simulink model "NoLineal_Linealizado"  (R2019a)
settings: Solver=ode4  StartTime=0.0  StopTime=0.6  FixedStep=0.001  RelTol=1e-3  EnableMultiTasking=on
settings Model: Creator=Ezequiel  LastModifiedBy=ARLUBER1
settings DataIOCC: LimitDataPoints=on  SaveFormat=Array  ReturnWorkspaceOutputs=off
settings OptimizationCC: LifeSpan=inf
settings DebuggingCC: PregeneratedLibrarySubsystemCodeDiagnostic=none  SFUnexpectedBacktrackingDiag=warning  SFNoUnconditionalDefaultTransitionDiag=warning  SFExecutionAtInitializationDiag=none  ArithmeticOperatorsInVariantConditions=warning
settings HardwareCC: ProdBitPerPointer=32  ProdBitPerSizeT=32  ProdBitPerPtrDiffT=32  ProdLargestAtomicFloat=None  ProdIntDivRoundTo=Undefined  ProdEndianess=Unspecified  ProdWordSize=32  ProdHWDeviceType=32-bit Generic
settings ModelReferenceCC: PropagateSignalLabelsOutOfModel=off
settings SFSimCC: SimUseLocalCustomCode=off
settings RTWCC: RTWUseLocalCustomCode=off
settings CodeAppCC: StateflowObjectComments=on
settings GRTTargetCC: TargetLangStandard=C89/C90 (ANSI)  GeneratePreprocessorConditionals=Disable all
settings ConfigComp: CovMetricSettings=dw  CovHtmlReporting=on  CovSaveCumulativeToWorkspaceVar=on  CovSaveSingleToWorkspaceVar=on  CovExternalEMLEnable=off

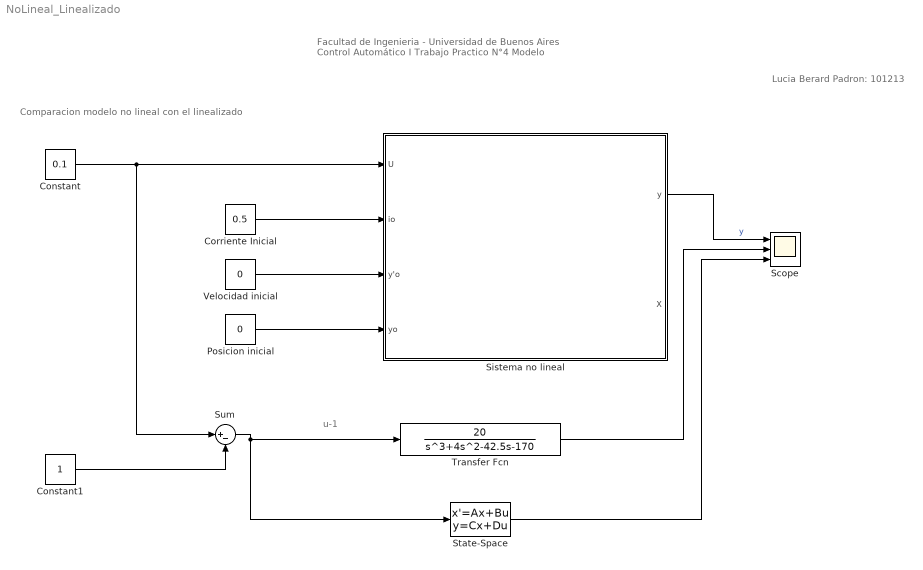
== system NoLineal_Linealizado ==
  note: Facultad de Ingenieria - Universidad de Buenos Aires
      | Control Automático I
      | Trabajo Practico N°4
      | Modelo
  note: Lucia Berard
      | Padron: 101213
  note: Comparacion modelo no lineal con el linealizado
  note: u-1
  Constant : Constant  Value=0.1
  Constant1 : Constant
  Corriente Inicial : Constant  Value=0.5
  Posicion inicial : Constant  Value=0
  Scope : Scope  NumInputPorts=3
  Sistema no lineal : Subsystem
  "State-Space " : StateSpace  A=[0 1 0;42.5 0 20;0 0 -4]  B=[0 0 1]'  C=[1 0 0]  D=0  InitialCondition=0
  Sum : Sum  Inputs=|+-
  Transfer Fcn : TransferFcn  Numerator=[20]  Denominator=[1 4 -42.5 -170]
  Velocidad inicial : Constant  Value=0
  wires:
  Corriente Inicial/1 -> Sistema no lineal/2(io)
  Velocidad inicial/1 -> Sistema no lineal/3(y'o)
  Posicion inicial/1 -> Sistema no lineal/4(yo)
  Constant/1 -> Sum/1, Sistema no lineal/1(U)
  Constant1/1 -> Sum/2
  Sum/1 -> "State-Space "/1, Transfer Fcn/1
  "State-Space "/1 -> Scope/3
  Sistema no lineal/1("y ") -> Scope/1  "y"
  Transfer Fcn/1 -> Scope/2

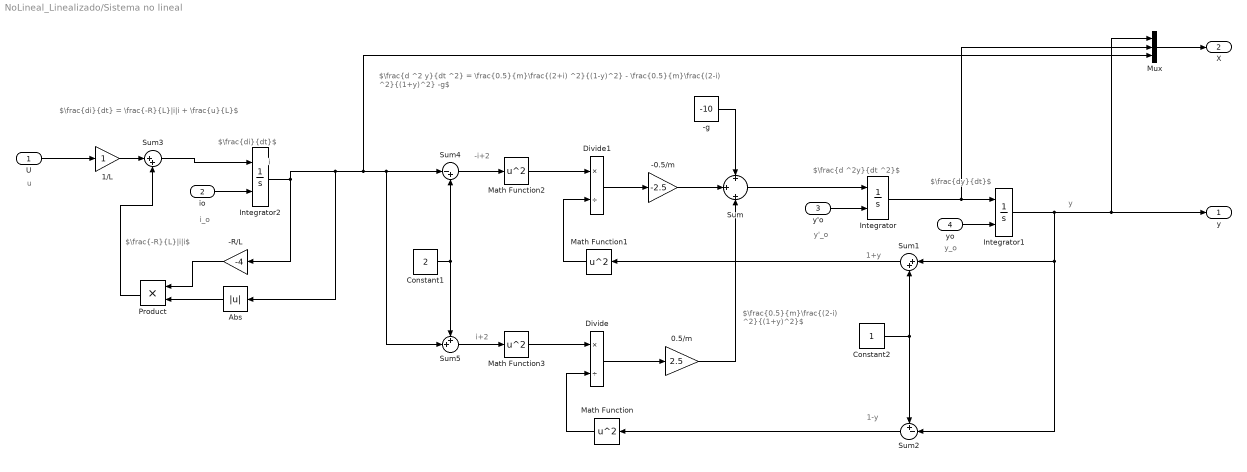
== system NoLineal_Linealizado/Sistema no lineal ==
  note: y_o
  note: y'_o
  note: i_o
  note: u
  note: i+2
  note: 1+y
  note: -i+2
  note: i
  note: y
  note: 1-y
  note: $\frac{di}{dt} = \frac{-R}{L}|i|i + \frac{u}{L}$
  note: $\frac{d ^2 y}{dt ^2} = \frac{0.5}{m}\frac{(2+i) ^2}{(1-y)^2} - \frac{0.5}{m}\frac{(2-i) ^2}{(1+y)^2} -g$
  note: $\frac{dy}{dt}$
  note: $\frac{d ^2y}{dt ^2}$
  note: $\frac{di}{dt}$
  note: $\frac{-R}{L}|i|i$
  note: $\frac{0.5}{m}\frac{(2-i) ^2}{(1+y)^2}$
  U : Inport  OutDataTypeStr=double
  io : Inport  Port=2  OutDataTypeStr=double
  y'o : Inport  Port=3
  yo : Inport  Port=4
  -0.5/m : Gain  Gain=-2.5
  -R/L : Gain  Gain=-4
  -g : Constant  Value=-10
  0.5/m : Gain  Gain=2.5
  1/L : Gain
  Abs : Abs
  Constant1 : Constant  Value=2
  Constant2 : Constant
  Divide : Product  Inputs=*/
  Divide1 : Product  Inputs=*/
  Integrator : Integrator  InitialConditionSource=external
  Integrator1 : Integrator  InitialConditionSource=external  UpperSaturationLimit=1  LowerSaturationLimit=-1
  Integrator2 : Integrator  InitialConditionSource=external
  Math Function{,1..3} (4 alike) : Math  Operator=square  SaturateOnIntegerOverflow=on
  Mux : Mux  Inputs=3
  Product : Product
  Sum : Sum  Inputs=+|+|+
  Sum1 : Sum  Inputs=|++
  Sum2 : Sum  Inputs=+-|
  Sum3 : Sum  Inputs=|++
  Sum4 : Sum  Inputs=|-+
  Sum5 : Sum  Inputs=++|
  "y " : Outport
  X : Outport  Port=2
  wires:
  Divide/1 -> 0.5/m/1
  Integrator2/1 -> Mux/3, Sum5/2, Sum4/1, Abs/1, -R/L/1
  Math Function2/1 -> Divide1/1
  Sum/1 -> Integrator/1
  io/1 -> Integrator2/2
  U/1 -> 1/L/1
  -R/L/1 -> Product/1
  Sum2/1 -> Math Function/1
  Sum1/1 -> Math Function1/1
  Sum5/1 -> Math Function3/1
  Sum4/1 -> Math Function2/1
  Integrator/1 -> Mux/2, Integrator1/1
  Math Function1/1 -> Divide1/2
  Divide1/1 -> -0.5/m/1
  Constant1/1 -> Sum4/2, Sum5/1
  -0.5/m/1 -> Sum/2
  Math Function/1 -> Divide/2
  0.5/m/1 -> Sum/3
  Math Function3/1 -> Divide/1
  Sum3/1 -> Integrator2/1
  -g/1 -> Sum/1
  Integrator1/1 -> Mux/1, "y "/1, Sum1/1, Sum2/2
  Constant2/1 -> Sum2/1, Sum1/2
  y'o/1 -> Integrator/2
  yo/1 -> Integrator1/2
  Mux/1 -> X/1
  1/L/1 -> Sum3/1
  Abs/1 -> Product/2
  Product/1 -> Sum3/2
